simulink model "H5_new"  (Simulink 9.2)
settings: Solver=ode45  StartTime=0.0  StopTime=2  RelTol=1e-3  EnableMultiTasking=on
undefined symbols (not defined in the file): dEgdT, EgRef, gcbh, k1, Rsh_array5pc, sps_rtmsupport, Tref_K, Ts_Control, VT_ref
libraries: powerlib x39, spsPVarrayModel x3, powerlib_meascontrol x1, simulink x1, simulink_extras x1
(part 1 of 6)
settings Model: Creator=Prince  LastModifiedBy=Aislyn VLSI-DSP
settings OptimizationCC: ExpressionDepthLimit=2147483647
settings DebuggingCC: SolverPrmCheckMsg=warning
settings GRTTargetCC: CombineOutputUpdateFcns=on  GRTInterface=off
settings SimscapeCC: SimscapeNormalizeSystem=off

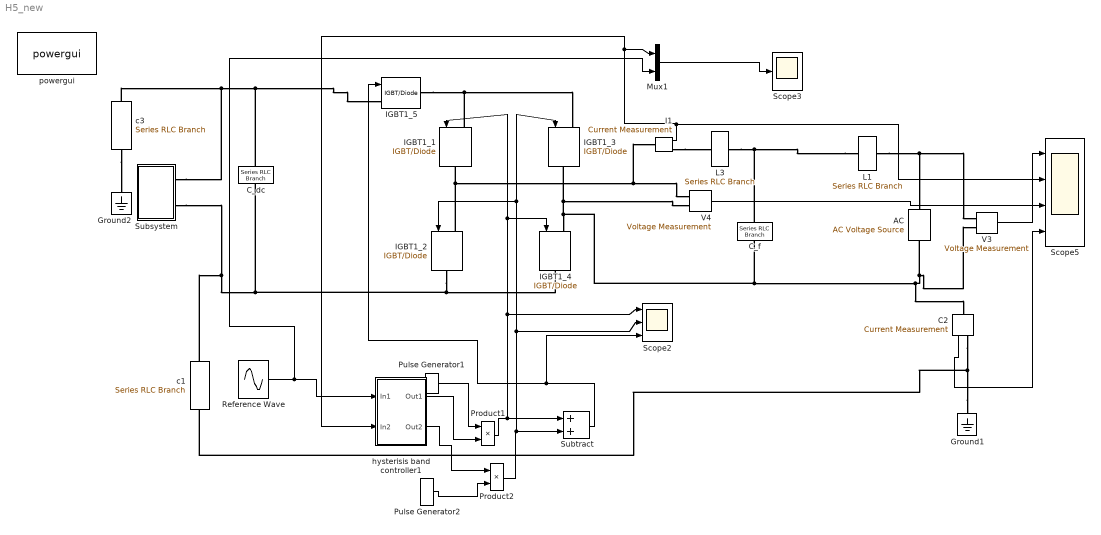
== system H5_new ==
  AC : powerlib/Electrical Sources/AC Voltage Source  Amplitude=220  Phase=0  Frequency=50  SampleTime=0  Measurements=Voltage  BusType=swing  Pref=10e3  Qref=0  Qmin=-inf  Qmax=+inf
      settings: SourceProductName=Simscape Electrical
  C2 : powerlib/Measurements/Current Measurement  PhasorSimulation=off  OutputType=Complex  PSBequivalent=0
      settings: SourceProductName=Simscape Electrical
  C_dc : powerlib/Elements/Series RLC Branch  LConnTagsString=__new0  RConnTagsString=__new0  BranchType=RC  Resistance=1e-3  Inductance=4e-3  SetiL0=off  InitialCurrent=0  Capacitance=250e-6  Setx0=off  InitialVoltage=0  Measurements=None
      settings: SourceProductName=Simscape Electrical
  C_f : powerlib/Elements/Series RLC Branch  LConnTagsString=__new0  RConnTagsString=__new0  BranchType=RC  Resistance=1e-3  Inductance=4e-3  SetiL0=off  InitialCurrent=0  Capacitance=3.45e-6  Setx0=off  InitialVoltage=0  Measurements=None
      settings: SourceProductName=Simscape Electrical
  Ground1 : powerlib/Elements/Ground  LConnTagsString=a
      settings: SourceProductName=Simscape Electrical
  Ground2 : powerlib/Elements/Ground  LConnTagsString=a
      settings: SourceProductName=Simscape Electrical
  I1 : powerlib/Measurements/Current Measurement  Tag=PoWeRsYsTeMmEaSuReMeNt  PhasorSimulation=off  OutputType=Magnitude  PSBequivalent=0
      settings: SourceProductName=Simscape Electrical
  IGBT1_{1..5} (5 alike) : powerlib/Power Electronics/IGBT//Diode  Ron=1e-3  Rs=1e5  Cs=inf  Measurements=off
      settings: SourceProductName=Simscape Electrical
  L1 : powerlib/Elements/Series RLC Branch  LConnTagsString=__new0  RConnTagsString=__new0  BranchType=RL  Resistance=1e-3  Inductance=5.7e-3  SetiL0=off  InitialCurrent=0  Capacitance=1e-6  Setx0=off  InitialVoltage=0  Measurements=None
      settings: SourceProductName=Simscape Electrical
  L3 : powerlib/Elements/Series RLC Branch  LConnTagsString=__new0  RConnTagsString=__new0  BranchType=RL  Resistance=1e-3  Inductance=17.7e-3  SetiL0=off  InitialCurrent=0  Capacitance=1e-6  Setx0=off  InitialVoltage=0  Measurements=None
      settings: SourceProductName=Simscape Electrical
  Mux1 : Mux  Inputs=2
  Product1 : Product  RndMeth=Zero
  Product2 : Product  RndMeth=Zero
  Pulse Generator1 : DiscretePulseGenerator  PulseType=Time based  Period=20e-3  PulseWidth=49.5
  Pulse Generator2 : DiscretePulseGenerator  PulseType=Time based  Period=20e-3  PulseWidth=49.5  PhaseDelay=10e-3
  Reference Wave : Sin  Amplitude=2  Frequency=2*pi*50  SampleTime=0
  Scope2 : Scope  NumInputPorts=3
  Scope3 : Scope
  Scope5 : Scope  NumInputPorts=4
  Subsystem : Subsystem
  Subtract : Sum
  V3 : powerlib/Measurements/Voltage Measurement  PhasorSimulation=off  OutputType=Complex  PSBequivalent=0
      settings: SourceProductName=Simscape Electrical
  V4 : powerlib/Measurements/Voltage Measurement  PhasorSimulation=off  OutputType=Complex  PSBequivalent=0
      settings: SourceProductName=Simscape Electrical
  c1 : powerlib/Elements/Series RLC Branch  LConnTagsString=__new0  RConnTagsString=__new0  BranchType=RC  Resistance=11.2  Inductance=1e-3  SetiL0=off  InitialCurrent=0  Capacitance=100e-9  Setx0=off  InitialVoltage=0  Measurements=None
      settings: SourceProductName=Simscape Electrical
  c3 : powerlib/Elements/Series RLC Branch  LConnTagsString=__new0  RConnTagsString=__new0  BranchType=RC  Resistance=11.2  Inductance=1e-3  SetiL0=off  InitialCurrent=0  Capacitance=100e-9  Setx0=off  InitialVoltage=0  Measurements=None
      settings: SourceProductName=Simscape Electrical
  hysterisis band controller1 : Subsystem
  powergui : powerlib/powergui  Priority=1  SimulationMode=Discrete  SampleTime=5e-6  frequency=60  Iterations=50  frequencyindice=0  Pbase=100e6  ErrMax=1e-4  UnitsV=kV  UnitsW=MW  buscounter=0  FunctionMessages=off  echomessages=off  EnableUseOfTLC=off  CurrentSourceSwitches=off  DisableSnubberDevices=off  DisableRonSwitches=off  DisableVfSwitches=off  DisplayEquations=off  SolverType=Tustin  Interpol=off  ExternalGateDelay=off  methode=off  Ts=0  x0status=blocks  SPID=off  SwTol=0  HookPort=off  RestoreLinks=warning  ResistiveCurrentMeasurement=off  Frange=[0:2:500]  Ylog=off  Xlog=on  ShowGrid=off  save=off  variable=ZData  structure=sps1phPWM1_str2  ZoomFFT=off  StartTime=0.02  cycles=2  DisplayStyle=1  fundamental=50  FreqAxis=off  MaxFrequency=100000  frequencyindicesteady=1  RmsSteady=1  display=off
  wires:
  C2/1 -> Scope5/4
  V4/1 -> Scope5/3
  V3/1 -> Scope5/1
  I1/1 -> Scope5/2, hysterisis band controller1/2(In2), Mux1/1
  Subtract/1 -> IGBT1_5/1, Scope2/3
  Product2/1 -> Subtract/2, IGBT1_3/1, IGBT1_2/1, Scope2/2
  Product1/1 -> Subtract/1, IGBT1_1/1, IGBT1_4/1, Scope2/1
  Mux1/1 -> Scope3/1
  Reference Wave/1 -> hysterisis band controller1/1(In1), Mux1/2
  Pulse Generator1/1 -> Product1/1
  Pulse Generator2/1 -> Product2/2
  hysterisis band controller1/2(Out2) -> Product2/1
  hysterisis band controller1/1(Out1) -> Product1/2
  connections:
  Subsystem/RConn2 -- c1/RConn1 -- IGBT1_4/RConn1 -- IGBT1_2/RConn1 -- C_dc/LConn1
  Ground1/LConn1 -- c1/LConn1 -- C2/RConn1
  L1/RConn1 -- AC/RConn1 -- V3/LConn1
  C_f/LConn1 -- IGBT1_3/RConn1 -- V4/LConn2 -- IGBT1_4/LConn1 -- C2/LConn1 -- AC/LConn1 -- V3/LConn2
  L1/LConn1 -- L3/RConn1 -- C_f/RConn1
  Subsystem/RConn1 -- c3/RConn1 -- C_dc/RConn1 -- IGBT1_5/LConn1
  IGBT1_5/RConn1 -- IGBT1_1/LConn1 -- IGBT1_3/LConn1
  IGBT1_2/LConn1 -- IGBT1_1/RConn1 -- V4/LConn1 -- I1/LConn1
  c3/LConn1 -- Ground2/LConn1
  I1/RConn1 -- L3/LConn1
